simulink model "DC_Motor_Model"  (Simulink 7.5)
settings: Solver=ode45  StartTime=0.0  StopTime=10.0  MaxStep=0.01  RelTol=1e-3
values from neighbouring files (symbols this model uses):
  B = [0 ... (first row only)    [system_eq.m]
  K = 0.01    [open_loop.m]    (also in pid_controller.m; system_eq.m)
settings Model: Creator=Victor  LastModifiedBy=Victor
settings OptimizationCC: InitFltsAndDblsToZero=on
settings DebuggingCC: SaveWithParameterizedLinksMsg=none  SignalResolutionControl=TryResolveAllWithWarning  MultiTaskDSMMsg=warning  MultiTaskCondExecSysMsg=none  StrictBusMsg=Warning
settings RTWCC: IncludeERTFirstTime=on
settings GRTTargetCC: TargetFcnLib=ansi_tfl_tmw.mat

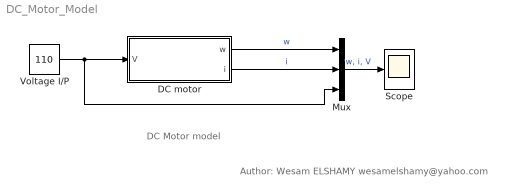
== system DC_Motor_Model ==
  note: DC Motor model
  note: Author: Wesam ELSHAMY
      | wesamelshamy@yahoo.com
  DC motor : Subsystem  mask(DC Motor){L=0.1, Kphi=0.3, J=0.1, b=0.01, R=2}
      mask help:
      | Takes the DC voltage as input, and outputs angular velocity (w) and current (i)
      | L => windings inductance		Kphi => emf constant
      | J => loads moment of inertial		b => viscous friction
      | R => windings resistance
      mask Display:
      | port_label('input', 1, 'V')
      | port_label('output', 2, 'i')
      | port_label('output', 1, 'w')
      | disp('DC Motor')
  Mux : Mux  Inputs=3
  Scope : Scope
      settings: TimeRange=10  YMin=0  YMax=400
  Voltage I/P : Constant  Value=110  OutDataType=sfix(16)  OutScaling=2^0
  wires:
  Voltage I/P/1 -> DC motor/1(V), Mux/3
  DC motor/1(w) -> Mux/1  "w"
  DC motor/2(i) -> Mux/2  "i"
  Mux/1 -> Scope/1  "w, i, V"

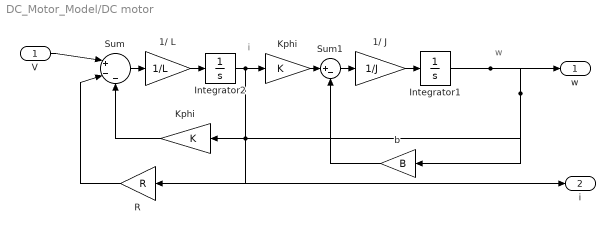
== system DC_Motor_Model/DC motor ==
  note: i
  note: w
  V : Inport  OutDataType=sfix(16)  OutScaling=2^0
  1/ J : Gain  Gain=1/J  ParameterDataType=sfix(16)  ParameterScaling=2^0  OutDataType=sfix(16)  OutScaling=2^0
  1/ L : Gain  Gain=1/L  ParameterDataType=sfix(16)  ParameterScaling=2^0  OutDataType=sfix(16)  OutScaling=2^0
  Integrator1 : Integrator
  Integrator2 : Integrator
  Kphi : Gain  Gain=K  ParameterDataType=sfix(16)  ParameterScaling=2^0  OutDataType=sfix(16)  OutScaling=2^0
  "Kphi " : Gain  Gain=K  ParameterDataType=sfix(16)  ParameterScaling=2^0  OutDataType=sfix(16)  OutScaling=2^0
  R : Gain  Gain=R  ParameterDataType=sfix(16)  ParameterScaling=2^0  OutDataType=sfix(16)  OutScaling=2^0
  Sum : Sum  Inputs=|+--  OutDataType=sfix(16)  OutScaling=2^0
  Sum1 : Sum  Inputs=|+-  OutDataType=sfix(16)  OutScaling=2^0
  b : Gain  Gain=B  ParameterDataType=sfix(16)  ParameterScaling=2^0  OutDataType=sfix(16)  OutScaling=2^0
  w : Outport  OutDataType=sfix(16)  OutScaling=2^0
  i : Outport  Port=2  OutDataType=sfix(16)  OutScaling=2^0
  wires:
  V/1 -> Sum/1
  Sum/1 -> 1/ L/1
  1/ L/1 -> Integrator2/1
  Integrator2/1 -> Kphi/1, R/1, i/1
  Kphi/1 -> Sum1/1
  Sum1/1 -> 1/ J/1
  1/ J/1 -> Integrator1/1
  Integrator1/1 -> "Kphi "/1, b/1, w/1
  b/1 -> Sum1/2
  "Kphi "/1 -> Sum/3
  R/1 -> Sum/2
